simulink model "Inverted_pendulum_model"  (R2023b)
settings: Solver=FixedStepAuto  StartTime=0.0  StopTime=inf  FixedStep=0.01  RelTol=1e-3
values from neighbouring files (symbols this model uses):
  b = 0.01    [PoleData150.mat]    (also in PoleParams1.mat = 0.00537612177045; estbmlLR_TRR.mat = 0.00681611435687; estimatemlbi.mat = 0.0059795291199; params.m)
  g = 9.81    [PendulumDirectionfield.m]    (also in PoleData150.mat; PoleParams1.mat = 9.78; estbmlLR_TRR.mat; estimatemlbi.mat)
  l = 0.514    [InitialCondition_exp_3.mat]    (also in InitialCondition_exp_6.mat; PendulumDirectionfield.m = 0.493; PoleData150.mat = 0.52; PoleParams1.mat = 0.5)
  m = 0.226    [InitialCondition_exp_3.mat]    (also in InitialCondition_exp_6.mat; PoleData150.mat = 0.093; PoleParams1.mat = 0.09216; estbmlLR_TRR.mat = 0.127471902163)
settings Model: Creator=tanawatp  LastModifiedBy=tanawatp
settings DataIOCC: OutputOption=AdditionalOutputTimes  OutputTimes=SDO_OutputTimes  ReturnWorkspaceOutputsName=SDOSimTest_Log

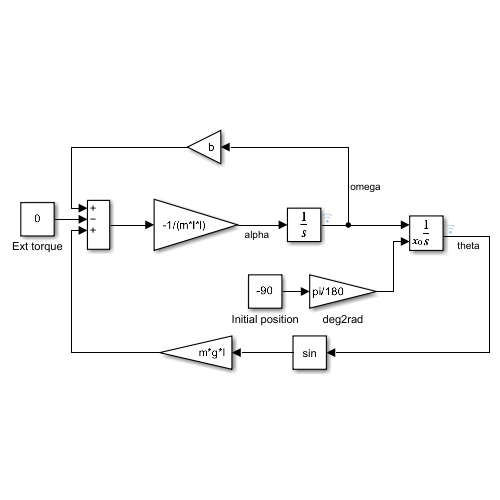
[thumbnail: Simulink's stored preview of the top-level diagram]
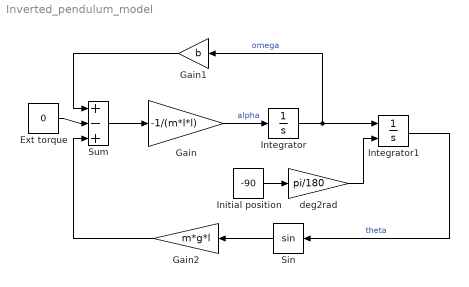
== system Inverted_pendulum_model ==
  Ext torque : Constant  Value=0
  Gain : Gain  Gain=-1/(m*l*l)  ParamDataTypeStr=double  OutDataTypeStr=double
  Gain1 : Gain  Gain=b
  Gain2 : Gain  Gain=m*g*l
  Initial position : Constant  Value=-90
  Integrator : Integrator
  Integrator1 : Integrator  InitialConditionSource=external  ContinuousStateAttributes='position'
  Sin : Trigonometry
  Sum : Sum  Inputs=+-+|
  deg2rad : Gain  Gain=pi/180
  wires:
  Ext torque/1 -> Sum/2
  Sum/1 -> Gain/1
  Gain/1 -> Integrator/1  "alpha"
  Integrator/1 -> Gain1/1, Integrator1/1  "omega"
  Gain1/1 -> Sum/1
  Initial position/1 -> deg2rad/1
  deg2rad/1 -> Integrator1/2
  Integrator1/1 -> Sin/1  "theta"
  Sin/1 -> Gain2/1
  Gain2/1 -> Sum/3
